simulink model "dc_engine_random_sig_random_period"  (R2019a)
settings: Solver=ode3  StartTime=0.0  StopTime=100  FixedStep=0.01  RelTol=1e-3
model workspace (MAT data in the model file):
  Kb = 0.01
  Kt = 0.001
  La = 0.5
  Ra = 1
settings Model: OrderedModelArguments=off  Creator=root  LastModifiedBy=root

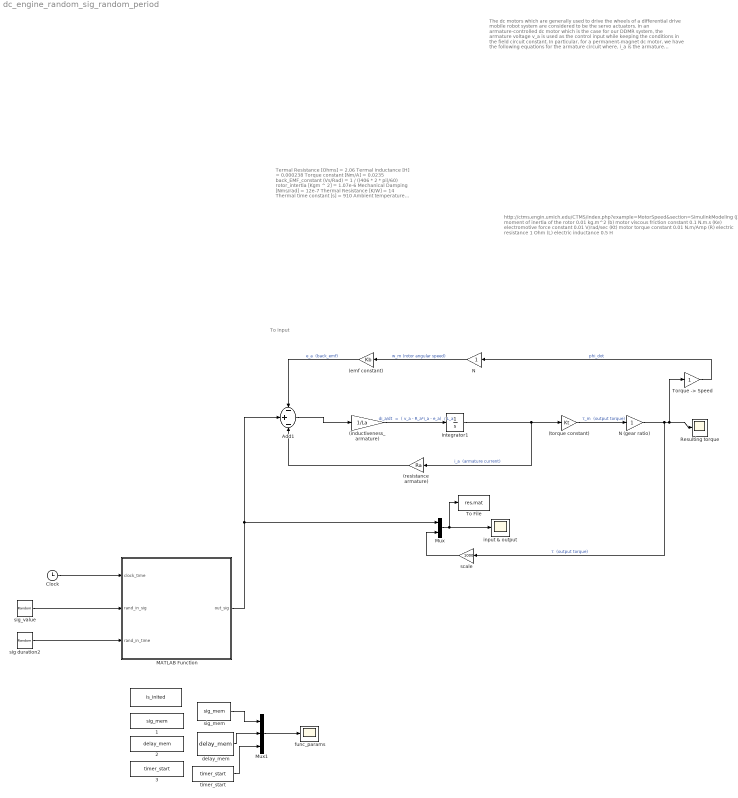
== system dc_engine_random_sig_random_period ==
  note: To input
  note: http://ctms.engin.umich.edu/CTMS/index.php?example=MotorSpeed&section=SimulinkModeling
      |
      | (J) moment of inertia of the rotor 0.01 kg.m^2
      | (b) motor viscous friction constant 0.1 N.m.s
      | (Ke) electromotive force constant 0.01 V/rad/sec
      | (Kt) motor torque constant 0.01 N.m/Amp
      | (R) electric resistance 1 Ohm
      | (L) electric inductance 0.5 H
  note: Termal Resistance [Ohms] = 2.06
      | Termal inductance [H] = 0.000238
      | Torque constant [Nm/A] = 0.0235
      | back_EMF_constant (Vs/Rad) = 1 / ((406 * 2 * pi)/60)
      | rotor_intertia [Kgm ^ 2] = 1.07e-6
      | Mechanical Damping [Nms/rad] = 12e-7
      | Thermal Resistance [K/W] = 14
      | Thermal time constant [s] = 910
      | Ambient temperature [C] = 22
  note: The dc motors which are generally used to drive the wheels of a differential drive mobile robot system are considered to be the servo actuators. In an armature-controlled dc motor which is the case for our DDMR system, the armature voltage v_a is used as the control input while keeping the conditions in the field circuit constant. In particular, for a permanent-magnet dc motor, we have the following equations for the armature circuit
      |
      | where, i_a is the armature current,(Ra ,La ) is the resistance and inductance of the armature winding respectively, e_a is the back emf, w_m is the rotor angular speed , τ_m is the motor torque, (Kt ,Kb ) are the torque constant and back emf constant respectively, N is the gear ratio, and is τ the output torque applied to the wheel.
      |
      | KD: Rewrite first as:
      | di_a/dt = ( v_a - R_a*i_a - e_a) / L_a
  " " : DataStoreMemory  DataStoreName=is_inited  ReadBeforeWriteMsg=warning  WriteAfterWriteMsg=warning  WriteAfterReadMsg=warning  InitialValue=false  ShowAdditionalParam=off  OutDataTypeStr=boolean
  " (inductiveness_armature)" : Gain  Gain=1/La
  " 1" : DataStoreMemory  DataStoreName=sig_mem  ReadBeforeWriteMsg=warning  WriteAfterWriteMsg=warning  WriteAfterReadMsg=warning  InitialValue=3  ShowAdditionalParam=off  OutDataTypeStr=double
  " 2" : DataStoreMemory  DataStoreName=delay_mem  ReadBeforeWriteMsg=warning  WriteAfterWriteMsg=warning  WriteAfterReadMsg=warning  ShowAdditionalParam=off  OutDataTypeStr=double
  " 3" : DataStoreMemory  DataStoreName=timer_start  ReadBeforeWriteMsg=warning  WriteAfterWriteMsg=warning  WriteAfterReadMsg=warning  ShowAdditionalParam=off  OutDataTypeStr=double
  (emf constant) : Gain  Gain=Kb
  (resistance armature) : Gain  Gain=Ra
  (torque constant) : Gain  Gain=Kt
  Add1 : Sum  Inputs=-+-
  Clock : Clock
  Integrator1 : Integrator
  MATLAB Function : MATLAB Function  TreatAsAtomicUnit=on
  Mux : Mux  Inputs=2
  Mux1 : Mux  Inputs=3
  N : Gain
  N (gear ratio) : Gain
  Resulting torque : Scope
  To File : ToFile  Filename=res.mat  SampleTime=0.01
  "Torque -> Speed " : Gain
  delay_mem : DataStoreRead  DataStoreName=delay_mem
  func_params : Scope
  input & output : Scope
  scale : Gain  Gain=1000
  sig duration2 : UniformRandomNumber  Minimum=4  Maximum=15  Seed=42  SampleTime=4
  "sig_mem " : DataStoreRead  DataStoreName=sig_mem
  sig_value : UniformRandomNumber  Minimum=8  Maximum=15  Seed=43  SampleTime=5
  timer_start : DataStoreRead  DataStoreName=timer_start
  wires:
  N (gear ratio)/1 -> "Torque -> Speed "/1, Resulting torque/1, scale/1  "τ  (output torque)"
  (torque constant)/1 -> N (gear ratio)/1  "τ_m  (output torque)"
  (emf constant)/1 -> Add1/1  "e_a  (back_emf)"
  N/1 -> (emf constant)/1  "w_m (rotor angular speed)"
  "Torque -> Speed "/1 -> N/1  "phi_dot"
  Add1/1 -> " (inductiveness_armature)"/1
  Integrator1/1 -> (resistance armature)/1, (torque constant)/1  "i_a  (armature current)"
  (resistance armature)/1 -> Add1/3
  " (inductiveness_armature)"/1 -> Integrator1/1  "di_a/dt  =  ( v_a - R_a*i_a - e_a)  / L_a"
  Mux/1 -> To File/1, input & output/1
  Clock/1 -> MATLAB Function/1(clock_time)
  sig_value/1 -> MATLAB Function/2(rand_in_sig)
  sig duration2/1 -> MATLAB Function/3(rand_in_time)
  "sig_mem "/1 -> Mux1/1
  delay_mem/1 -> Mux1/2
  timer_start/1 -> Mux1/3
  Mux1/1 -> func_params/1
  MATLAB Function/1(out_sig) -> Add1/2, Mux/1
  scale/1 -> Mux/2

== matlab function dc_engine_random_sig_random_period/MATLAB Function ==
  settings: updateMethod=DISCRETE
  data: clock_time input; out_sig output; rand_in_sig input; rand_in_time input; sig_mem data_store_memory; delay_mem data_store_memory; is_inited data_store_memory; timer_start data_store_memory
function out_sig  = randomize_time_period(clock_time, rand_in_sig, rand_in_time)
global sig_mem;
global delay_mem;
global is_inited;
global timer_start;
if (~is_inited)
    is_inited = true;
    timer_start = clock_time;
    sig_mem = rand_in_sig;
    delay_mem = rand_in_time;
end

if (clock_time - timer_start ) > delay_mem
    timer_start = clock_time;
    sig_mem = rand_in_sig;
    delay_mem = rand_in_time;
end

out_sig = sig_mem;
